simulink model "pid_tunning"  (R2018b)
settings: Solver=VariableStepAuto  StartTime=0.0  StopTime=50  RelTol=1e-3
settings Model: Creator=arthus  LastModifiedBy=arthus

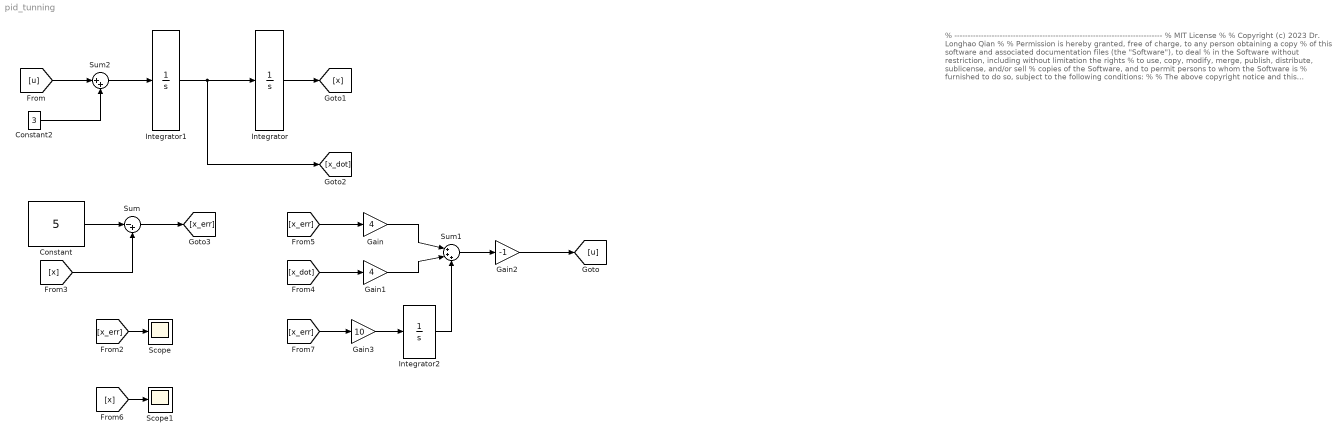
== system pid_tunning ==
  note: % ------------------------------------------------------------------------------
      | % MIT License
      | %
      | % Copyright (c) 2023 Dr. Longhao Qian
      | %
      | % Permission is hereby granted, free of charge, to any person obtaining a copy
      | % of this software and associated documentation files (the "Software"), to deal
      | % in the Software without restriction, including without limitation the rights
      | % to use, copy, modify, merge, publish, distribute, sublicense, and/or sell
      | % copies of the Software, and to permit persons to whom the Software is
      | % furnished to do so, subject to the following conditions:
      | %
      | % The above copyright notice and this permission notice shall be included in all
      | % copies or substantial portions of the Software.
      | %
      | % THE SOFTWARE IS PROVIDED "AS IS", WITHOUT WARRANTY OF ANY KIND, EXPRESS OR
      | % IMPLIED, INCLUDING BUT NOT LIMITED TO THE WARRANTIES OF MERCHANTABILITY,
      | % FITNESS FOR A PARTICULAR PURPOSE AND NONINFRINGEMENT. IN NO EVENT SHALL THE
      | % AUTHORS OR COPYRIGHT HOLDERS BE LIABLE FOR ANY CLAIM, DAMAGES OR OTHER
      | % LIABILITY, WHETHER IN AN ACTION OF CONTRACT, TORT OR OTHERWISE, ARISING FROM,
      | % OUT OF OR IN CONNECTION WITH THE SOFTWARE OR THE USE OR OTHER DEALINGS IN THE
      | % SOFTWARE.
      | % ------------------------------------------------------------------------------
  Constant : Constant  Value=5
  Constant2 : Constant  Value=3
  Gain : Gain  Gain=4
  Gain1 : Gain  Gain=4
  Gain2 : Gain  Gain=-1
  Gain3 : Gain  Gain=10
  Integrator : Integrator
  Integrator1 : Integrator
  Integrator2 : Integrator
  Scope : Scope
  Scope1 : Scope
  Sum : Sum  Inputs=|-+
  Sum1 : Sum  Inputs=|+++
  Sum2 : Sum  Inputs=|++
  wires:
  Integrator/1 -> [x]
  Integrator1/1 -> [x_dot], Integrator/1
  Constant/1 -> Sum/1
  [x] -> Sum/2
  Sum/1 -> [x_err]
  [x_err] -> Gain/1
  Gain/1 -> Sum1/1
  Sum1/1 -> Gain2/1
  Gain2/1 -> [u]
  [x_err] -> Scope/1
  [x] -> Scope1/1
  [u] -> Sum2/1
  Sum2/1 -> Integrator1/1
  Constant2/1 -> Sum2/2
  [x_dot] -> Gain1/1
  Gain1/1 -> Sum1/2
  Gain3/1 -> Integrator2/1
  [x_err] -> Gain3/1
  Integrator2/1 -> Sum1/3
